simulink model "model"  (R2017a)
settings: Solver=ode4  StartTime=0.0  StopTime=100.0  FixedStep=0.01  RelTol=1e-3
values from neighbouring files (symbols this model uses):
  A = [k1+k2 -k2 0; -k2 k2+k3 -k3; 0 -k3 k3]    [Takietam.m]
  B = [1;0;0]    [Takietam.m]
  F = [c1+c2 -c2 0; -c2 c2+c3 -c3; 0 -c3 c3]    [Takietam.m]
  x0 = 0    [Takietam.m]
  xd0 = 0    [Takietam.m]
settings Model: Creator=LPA2  LastModifiedBy=LPA2

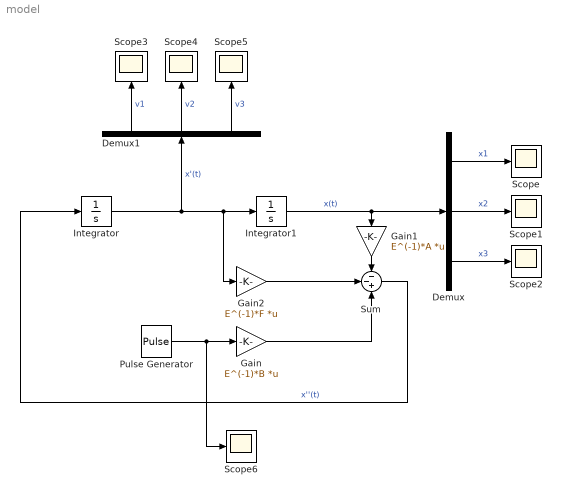
== system model ==
  Demux : Demux  Outputs=3
  Demux1 : Demux  Outputs=3
  Gain : Gain  Gain=E^(-1)*B  Multiplication=Matrix(K*u)
  Gain1 : Gain  Gain=E^(-1)*A  Multiplication=Matrix(K*u)
  Gain2 : Gain  Gain=E^(-1)*F  Multiplication=Matrix(K*u)
  Integrator : Integrator  InitialCondition=xd0
  Integrator1 : Integrator  InitialCondition=x0
  Pulse Generator : DiscretePulseGenerator  PulseType=Time based  Period=100
  Scope{,1..6} (7 alike) : Scope
  Sum : Sum  Inputs=--+
  wires:
  Integrator1/1 -> Demux/1, Gain1/1  "x(t)"
  Gain1/1 -> Sum/1
  Integrator/1 -> Gain2/1, Integrator1/1, Demux1/1  "x'(t)"
  Gain2/1 -> Sum/2
  Sum/1 -> Integrator/1  "x''(t)"
  Gain/1 -> Sum/3
  Demux/3 -> Scope2/1  "x3"
  Demux/2 -> Scope1/1  "x2"
  Demux/1 -> Scope/1  "x1"
  Demux1/1 -> Scope3/1  "v1"
  Demux1/2 -> Scope4/1  "v2"
  Demux1/3 -> Scope5/1  "v3"
  Pulse Generator/1 -> Scope6/1, Gain/1
